simulink model "pathNavigation_PID_start"  (R2017a)
settings: Solver=FixedStepDiscrete  StartTime=0.0  StopTime=inf  FixedStep=0.01  RelTol=1e-3
PreLoadFcn:
  | robotParameters;
  | load examplePathNavigationMap.mat;
undefined symbols (not defined in the file or in its folder): axleLength, motorIp, motorSp, ticksPerRot, wheelR
libraries: mobileRoboticsTrainingLib x7, simulink_extras x1
settings Model: Creator=sseshadr  LastModifiedBy=shiremat

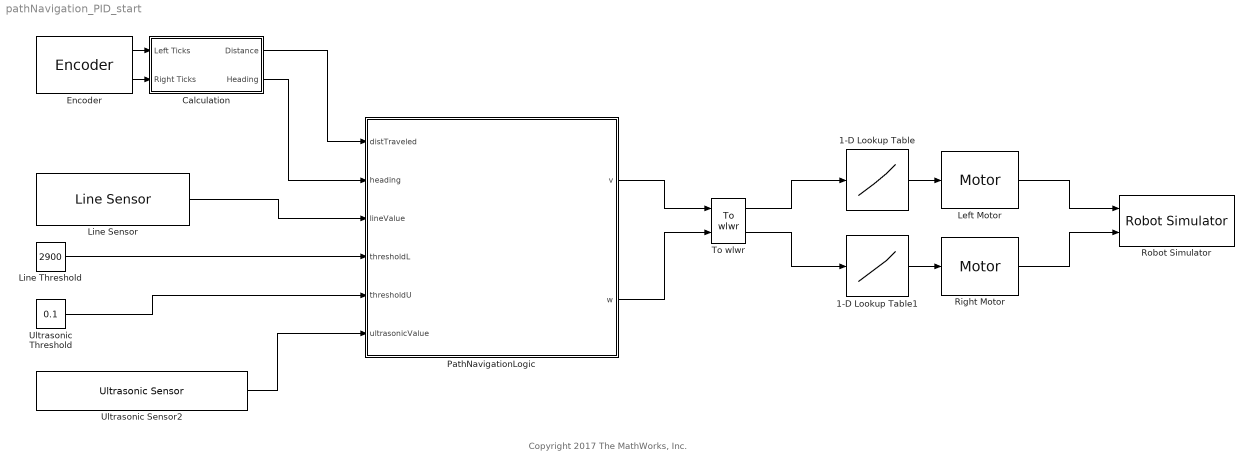
== system pathNavigation_PID_start ==
  note: Copyright 2017 The MathWorks, Inc.
  1-D Lookup Table : Lookup_n-D  NumberOfTableDimensions=1  BreakpointsForDimension1=motorSp  Table=motorIp  ExtrapMethod=Clip  InternalRulePriority=Speed  RndMeth=Simplest  InputSameDT=on
  1-D Lookup Table1 : Lookup_n-D  NumberOfTableDimensions=1  BreakpointsForDimension1=motorSp  Table=motorIp  ExtrapMethod=Clip  InternalRulePriority=Speed  RndMeth=Simplest  InputSameDT=on
  Calculation : Subsystem
  Encoder : mobileRoboticsTrainingLib/Encoder  axleLength=axleLength  wheelR=wheelR  ticksPerRot=ticksPerRot
      settings: SourceProductName=Mobile Robotics Training Library
  Left Motor : mobileRoboticsTrainingLib/Motor  motorPlant=wheelMotorModel  sensorType=Speed
      settings: SourceProductName=Mobile Robotics Training Library
  Line Sensor : mobileRoboticsTrainingLib/Line Sensor  mapVariable=mapForSim  envVal=2850  lineVal=2950  sensOff=[0.01 -0.01;0.01 0;0.01 0.01]
      settings: SourceProductName=Mobile Robotics Training Library
  Line Threshold : Constant  Value=2900
  PathNavigationLogic : Stateflow chart  TreatAsAtomicUnit=on
  Right Motor : mobileRoboticsTrainingLib/Motor  motorPlant=wheelMotorModel  sensorType=Speed
      settings: SourceProductName=Mobile Robotics Training Library
  Robot Simulator : mobileRoboticsTrainingLib/Robot Simulator  Priority=99  mapVar=mapForSim  startX=0.5  startY=0.25  startTheta=90  axleLength=axleLength  wheelR=wheelR
  To wlwr : mobileRoboticsTrainingLib/To wlwr  axleLength=axleLength  wheelR=wheelR
  Ultrasonic Sensor2 : mobileRoboticsTrainingLib/Ultrasonic Sensor  mapVar=mapForSim  maxSenRange=0.25  minSenRange=0.02  senRes=0.01  sensOff=[0 0]
      settings: SourceProductName=Mobile Robotics Training Library
  Ultrasonic Threshold : Constant  Value=0.1
  wires:
  Left Motor/1 -> Robot Simulator/1
  1-D Lookup Table1/1 -> Right Motor/1
  1-D Lookup Table/1 -> Left Motor/1
  Right Motor/1 -> Robot Simulator/2
  To wlwr/1 -> 1-D Lookup Table/1
  To wlwr/2 -> 1-D Lookup Table1/1
  PathNavigationLogic/1(v) -> To wlwr/1
  PathNavigationLogic/2(w) -> To wlwr/2
  Ultrasonic Sensor2/1 -> PathNavigationLogic/6(ultrasonicValue)
  Line Sensor/1 -> PathNavigationLogic/3(lineValue)
  Encoder/2 -> Calculation/2(Right Ticks)
  Encoder/1 -> Calculation/1(Left Ticks)
  Calculation/1(Distance) -> PathNavigationLogic/1(distTraveled)
  Calculation/2(Heading) -> PathNavigationLogic/2(heading)
  Line Threshold/1 -> PathNavigationLogic/4(thresholdL)
  Ultrasonic Threshold/1 -> PathNavigationLogic/5(thresholdU)

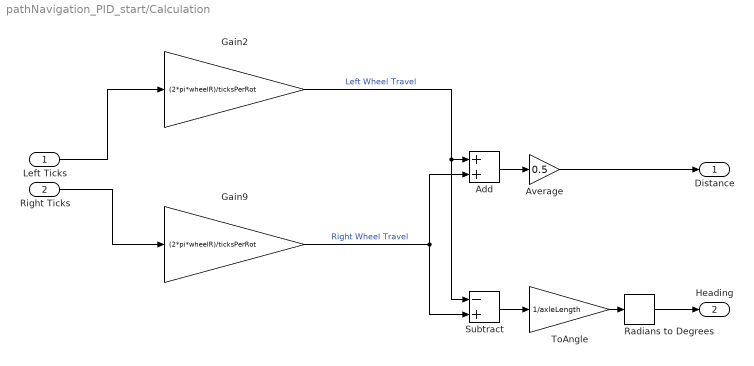
== system pathNavigation_PID_start/Calculation ==
  Left Ticks : Inport
  Right Ticks : Inport  Port=2
  Add : Sum
  Average : Gain  Gain=0.5
  Gain2 : Gain  Gain=(2*pi*wheelR)/ticksPerRot
  Gain9 : Gain  Gain=(2*pi*wheelR)/ticksPerRot
  Radians to Degrees : simulink_extras/Transformations/Radians to Degrees
  Subtract : Sum  Inputs=-+
  ToAngle : Gain  Gain=1/axleLength
  Distance : Outport
  Heading : Outport  Port=2
  wires:
  Average/1 -> Distance/1
  Add/1 -> Average/1
  Gain2/1 -> Subtract/1, Add/1  "Left Wheel Travel"
  Right Ticks/1 -> Gain9/1
  Left Ticks/1 -> Gain2/1
  Gain9/1 -> Subtract/2, Add/2  "Right Wheel Travel"
  Subtract/1 -> ToAngle/1
  ToAngle/1 -> Radians to Degrees/1
  Radians to Degrees/1 -> Heading/1

== stateflow chart pathNavigation_PID_start/PathNavigationLogic ==
  state SegmentA
    state MoveForward
      entry:
      v = 0.5;
    state Stop
      entry:
      v = 0;
    state Rotate
      entry:
      w = -1;
    state Stop1
      entry:
      w = 0;
    (default) -> SegmentA.MoveForward : %Start Dead Reckoning
    SegmentA.MoveForward -> SegmentA.Stop : [distTraveled >= 1.05]
    SegmentA.Stop -> SegmentA.Rotate
    SegmentA.Rotate -> SegmentA.Stop1 : [heading <= -90]
  state SegmentB
    state FindLine
      entry:
      v = 0.05;
    state GoLeft
      entry:
      v = 0.1;
      w = 1;
    state GoRight
      entry:
      v = 0.1;
      w = -1;
    state Stop
      entry:
      v = 0;
      w = 0;
    (default) -> FindLine
    FindLine -> GoLeft : [lineValue(2) > thresholdL]
    GoLeft -> GoRight [order 1] : [lineValue(2) < thresholdL]
    GoRight -> GoLeft [order 1] : [lineValue(2) >= thresholdL]
    GoLeft -> SegmentB.Stop [order 2] : [all(lineValue > thresholdL)]
    GoRight -> SegmentB.Stop [order 2] : [all(lineValue > thresholdL)]
  state SegmentC1
    state MoveForward
      entry:
      v = 0.5;
      currDist = distTraveled;
    state Stop
      entry:
      v = 0;
    state Rotate
      entry:
      w = 1;
      currHead = heading;
    state Stop1
      entry:
      w = 0;
    (default) -> SegmentC1.MoveForward : %Start Dead Reckoning
    SegmentC1.MoveForward -> SegmentC1.Stop : [distTraveled - currDist >= 0.2]
    SegmentC1.Stop -> SegmentC1.Rotate
    SegmentC1.Rotate -> SegmentC1.Stop1 : [heading - currHead >= 45]
  state SegmentD
    state Go
      entry: v = 0.2;
    state Stop
      entry: v = 0;
    (default) -> Go
    Go -> SegmentD.Stop : [(ultrasonicValue <= thresholdU) && (ultrasonicValue > 0)]
  (default) -> SegmentA
  SegmentA.Stop1 -> SegmentB
  SegmentB.Stop -> SegmentC1
  SegmentC1.Stop1 -> SegmentD
  data: distTraveled input; heading input; lineValue input; thresholdL input; thresholdU input; ultrasonicValue input; v output; w output; currDist local; currHead local
